simulink model "Milestone_2"  (R2020a)
settings: Solver=VariableStepAuto  StartTime=0.0  StopTime=3  RelTol=1e-3
libraries: simulink x10
settings Model: Creator=michk  LastModifiedBy=matthewterblanche

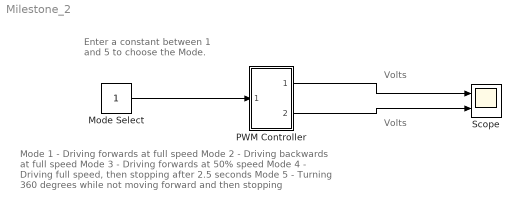
== system Milestone_2 ==
  note: Mode 1 - Driving forwards at full speed
      |
      | Mode 2 - Driving backwards at full speed
      |
      | Mode 3 - Driving forwards at 50% speed
      |
      | Mode 4 - Driving full speed, then stopping after 2.5 seconds
      |
      | Mode 5 - Turning 360 degrees while not moving forward and 			 then stopping
  note: Enter a constant between 1 and 5 to choose the Mode.
  note: Volts
  note: Volts
  Mode Select : Constant
  PWM Controller : Subsystem
  Scope : Scope  NumInputPorts=2
  wires:
  PWM Controller/2(Out2) -> Scope/2
  Mode Select/1 -> PWM Controller/1(In1)
  PWM Controller/1(Out1) -> Scope/1

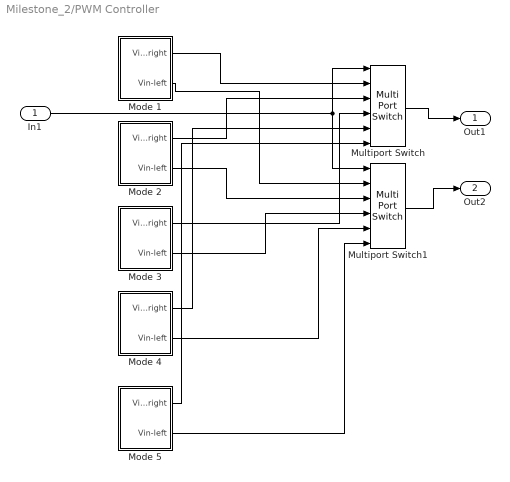
== system Milestone_2/PWM Controller ==
  In1 : Inport
  Mode 1 : Subsystem
  Mode 2 : Subsystem
  Mode 3 : Subsystem
  Mode 4 : Subsystem
  Mode 5 : Subsystem
  Multiport Switch : MultiPortSwitch  Inputs=5
  Multiport Switch1 : MultiPortSwitch  Inputs=5
  Out1 : Outport
  Out2 : Outport  Port=2
  wires:
  Multiport Switch/1 -> Out1/1
  Multiport Switch1/1 -> Out2/1
  In1/1 -> Multiport Switch/1, Multiport Switch1/1
  Mode 2/2(Vin-left) -> Multiport Switch1/3
  Mode 3/1(Vin-right) -> Multiport Switch/4
  Mode 5/2(Vin-left) -> Multiport Switch1/6
  Mode 4/1(Vin-right) -> Multiport Switch/5
  Mode 5/1(Vin-right) -> Multiport Switch/6
  Mode 2/1(Vin-right) -> Multiport Switch/3
  Mode 1/1(Vin-right) -> Multiport Switch/2
  Mode 1/2(Vin-left) -> Multiport Switch1/2
  Mode 4/2(Vin-left) -> Multiport Switch1/5
  Mode 3/2(Vin-left) -> Multiport Switch1/4

== system Milestone_2/PWM Controller/Mode 1 ==
  Subsystem : Subsystem
  Subsystem1 : Subsystem
  Vin-right : Outport
  Vin-left : Outport  Port=2
  wires:
  Subsystem1/1(Vin-left) -> Vin-left/1
  Subsystem/1(Vin-right) -> Vin-right/1

== system Milestone_2/PWM Controller/Mode 2 ==
  Subsystem : Subsystem
  Subsystem1 : Subsystem
  Vin-right : Outport
  Vin-left : Outport  Port=2
  wires:
  Subsystem1/1(Vin-left) -> Vin-left/1
  Subsystem/1(Vin-right) -> Vin-right/1

== system Milestone_2/PWM Controller/Mode 3 ==
  Subsystem : Subsystem
  Subsystem1 : Subsystem
  Vin-right : Outport
  Vin-left : Outport  Port=2
  wires:
  Subsystem1/1(Vin-left) -> Vin-left/1
  Subsystem/1(Vin-right) -> Vin-right/1

== system Milestone_2/PWM Controller/Mode 4 ==
  note: Stop motor after 2.5s
  Constant : Constant  Value=0
  Product : Product
  Product1 : Product
  Subsystem : Subsystem
  Subsystem1 : Subsystem
  Transport Delay : TransportDelay  DelayTime=2.5  InitialOutput=1  BufferSize=25600
  Vin-right : Outport
  Vin-left : Outport  Port=2
  wires:
  Subsystem1/1(Vin-left) -> Product/2
  Subsystem/1(Vin-right) -> Product1/2
  Product/1 -> Vin-left/1
  Product1/1 -> Vin-right/1
  Transport Delay/1 -> Product/1, Product1/1
  Constant/1 -> Transport Delay/1

== system Milestone_2/PWM Controller/Mode 5 ==
  Constant : Constant  Value=0
  Product : Product
  Product1 : Product
  Subsystem : Subsystem
  Subsystem1 : Subsystem
  Time motor must be on : TransportDelay  DelayTime=(0.175*pi/0.75)  InitialOutput=1  BufferSize=8192
  Vin-right : Outport
  Vin-left : Outport  Port=2
  wires:
  Constant/1 -> Time motor must be on/1
  Time motor must be on/1 -> Product1/1, Product/1
  Subsystem/1(Vin-right) -> Product/2
  Product/1 -> Vin-right/1
  Subsystem1/1(Vin-left) -> Product1/2
  Product1/1 -> Vin-left/1

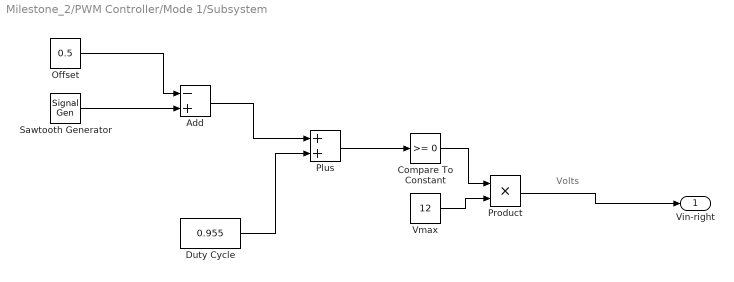
== system Milestone_2/PWM Controller/Mode 1/Subsystem ==
  note: Volts
  Add : Sum  Inputs=-+
  Compare To Constant : simulink/Logic and Bit Operations/Compare To Constant  relop=>=  const=0  OutDataTypeStr=boolean
  Duty Cycle : Constant  Value=0.955
  Offset : Constant  Value=0.5
  Plus : Sum
  Product : Product
  Sawtooth Generator : SignalGenerator  WaveForm=sawtooth  Amplitude=0.5  Frequency=10
  Vmax : Constant  Value=12
  Vin-right : Outport
  wires:
  Sawtooth Generator/1 -> Add/2
  Product/1 -> Vin-right/1
  Vmax/1 -> Product/2
  Duty Cycle/1 -> Plus/2
  Plus/1 -> Compare To Constant/1
  Offset/1 -> Add/1
  Compare To Constant/1 -> Product/1
  Add/1 -> Plus/1

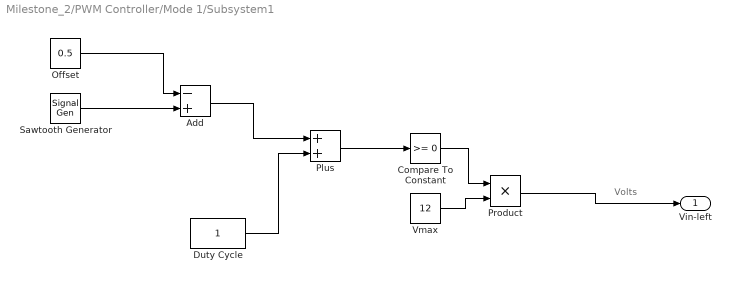
== system Milestone_2/PWM Controller/Mode 1/Subsystem1 ==
  note: Volts
  Add : Sum  Inputs=-+
  Compare To Constant : simulink/Logic and Bit Operations/Compare To Constant  relop=>=  const=0  OutDataTypeStr=boolean
  Duty Cycle : Constant
  Offset : Constant  Value=0.5
  Plus : Sum
  Product : Product
  Sawtooth Generator : SignalGenerator  WaveForm=sawtooth  Amplitude=0.5  Frequency=10
  Vmax : Constant  Value=12
  Vin-left : Outport
  wires:
  Sawtooth Generator/1 -> Add/2
  Product/1 -> Vin-left/1
  Vmax/1 -> Product/2
  Duty Cycle/1 -> Plus/2
  Plus/1 -> Compare To Constant/1
  Offset/1 -> Add/1
  Compare To Constant/1 -> Product/1
  Add/1 -> Plus/1

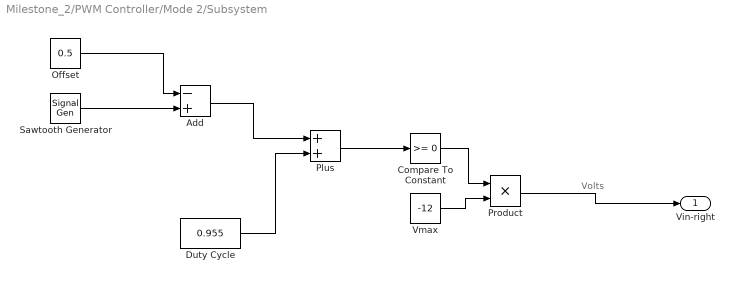
== system Milestone_2/PWM Controller/Mode 2/Subsystem ==
  note: Volts
  Add : Sum  Inputs=-+
  Compare To Constant : simulink/Logic and Bit Operations/Compare To Constant  relop=>=  const=0  OutDataTypeStr=boolean
  Duty Cycle : Constant  Value=0.955
  Offset : Constant  Value=0.5
  Plus : Sum
  Product : Product
  Sawtooth Generator : SignalGenerator  WaveForm=sawtooth  Amplitude=0.5  Frequency=10
  Vmax : Constant  Value=-12
  Vin-right : Outport
  wires:
  Sawtooth Generator/1 -> Add/2
  Product/1 -> Vin-right/1
  Vmax/1 -> Product/2
  Duty Cycle/1 -> Plus/2
  Plus/1 -> Compare To Constant/1
  Offset/1 -> Add/1
  Compare To Constant/1 -> Product/1
  Add/1 -> Plus/1

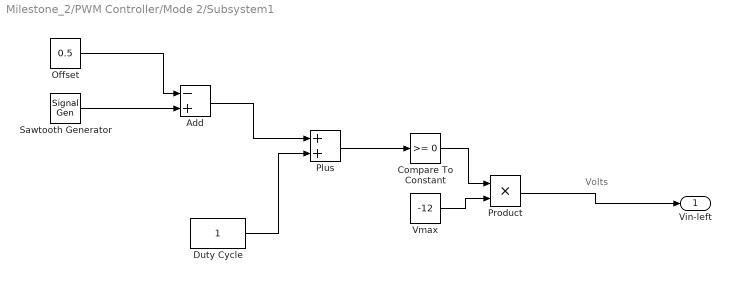
== system Milestone_2/PWM Controller/Mode 2/Subsystem1 ==
  note: Volts
  Add : Sum  Inputs=-+
  Compare To Constant : simulink/Logic and Bit Operations/Compare To Constant  relop=>=  const=0  OutDataTypeStr=boolean
  Duty Cycle : Constant
  Offset : Constant  Value=0.5
  Plus : Sum
  Product : Product
  Sawtooth Generator : SignalGenerator  WaveForm=sawtooth  Amplitude=0.5  Frequency=10
  Vmax : Constant  Value=-12
  Vin-left : Outport
  wires:
  Sawtooth Generator/1 -> Add/2
  Product/1 -> Vin-left/1
  Vmax/1 -> Product/2
  Duty Cycle/1 -> Plus/2
  Plus/1 -> Compare To Constant/1
  Offset/1 -> Add/1
  Compare To Constant/1 -> Product/1
  Add/1 -> Plus/1

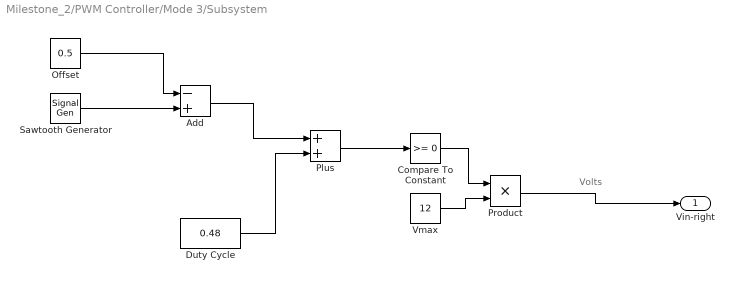
== system Milestone_2/PWM Controller/Mode 3/Subsystem ==
  note: Volts
  Add : Sum  Inputs=-+
  Compare To Constant : simulink/Logic and Bit Operations/Compare To Constant  relop=>=  const=0  OutDataTypeStr=boolean
  Duty Cycle : Constant  Value=0.48
  Offset : Constant  Value=0.5
  Plus : Sum
  Product : Product
  Sawtooth Generator : SignalGenerator  WaveForm=sawtooth  Amplitude=0.5  Frequency=10
  Vmax : Constant  Value=12
  Vin-right : Outport
  wires:
  Sawtooth Generator/1 -> Add/2
  Product/1 -> Vin-right/1
  Vmax/1 -> Product/2
  Duty Cycle/1 -> Plus/2
  Plus/1 -> Compare To Constant/1
  Offset/1 -> Add/1
  Compare To Constant/1 -> Product/1
  Add/1 -> Plus/1

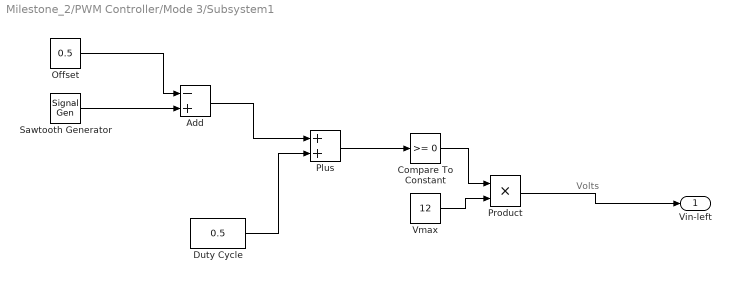
== system Milestone_2/PWM Controller/Mode 3/Subsystem1 ==
  note: Volts
  Add : Sum  Inputs=-+
  Compare To Constant : simulink/Logic and Bit Operations/Compare To Constant  relop=>=  const=0  OutDataTypeStr=boolean
  Duty Cycle : Constant  Value=0.5
  Offset : Constant  Value=0.5
  Plus : Sum
  Product : Product
  Sawtooth Generator : SignalGenerator  WaveForm=sawtooth  Amplitude=0.5  Frequency=10
  Vmax : Constant  Value=12
  Vin-left : Outport
  wires:
  Sawtooth Generator/1 -> Add/2
  Product/1 -> Vin-left/1
  Vmax/1 -> Product/2
  Duty Cycle/1 -> Plus/2
  Plus/1 -> Compare To Constant/1
  Offset/1 -> Add/1
  Compare To Constant/1 -> Product/1
  Add/1 -> Plus/1

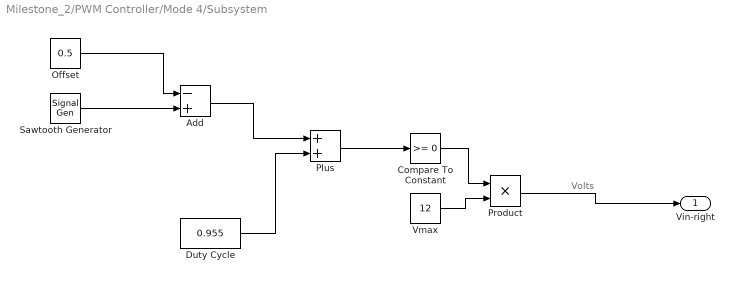
== system Milestone_2/PWM Controller/Mode 4/Subsystem ==
  note: Volts
  Add : Sum  Inputs=-+
  Compare To Constant : simulink/Logic and Bit Operations/Compare To Constant  relop=>=  const=0  OutDataTypeStr=boolean
  Duty Cycle : Constant  Value=0.955
  Offset : Constant  Value=0.5
  Plus : Sum
  Product : Product
  Sawtooth Generator : SignalGenerator  WaveForm=sawtooth  Amplitude=0.5  Frequency=10
  Vmax : Constant  Value=12
  Vin-right : Outport
  wires:
  Sawtooth Generator/1 -> Add/2
  Product/1 -> Vin-right/1
  Vmax/1 -> Product/2
  Duty Cycle/1 -> Plus/2
  Plus/1 -> Compare To Constant/1
  Offset/1 -> Add/1
  Compare To Constant/1 -> Product/1
  Add/1 -> Plus/1

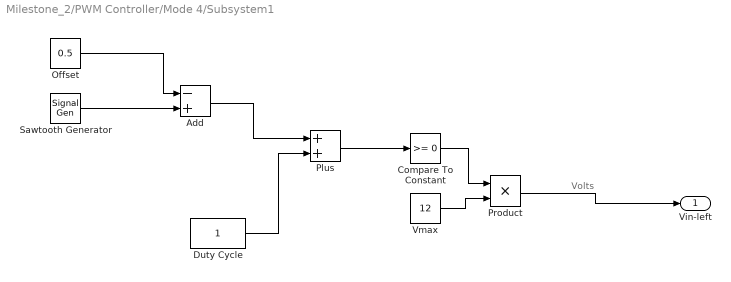
== system Milestone_2/PWM Controller/Mode 4/Subsystem1 ==
  note: Volts
  Add : Sum  Inputs=-+
  Compare To Constant : simulink/Logic and Bit Operations/Compare To Constant  relop=>=  const=0  OutDataTypeStr=boolean
  Duty Cycle : Constant
  Offset : Constant  Value=0.5
  Plus : Sum
  Product : Product
  Sawtooth Generator : SignalGenerator  WaveForm=sawtooth  Amplitude=0.5  Frequency=10
  Vmax : Constant  Value=12
  Vin-left : Outport
  wires:
  Sawtooth Generator/1 -> Add/2
  Product/1 -> Vin-left/1
  Vmax/1 -> Product/2
  Duty Cycle/1 -> Plus/2
  Plus/1 -> Compare To Constant/1
  Offset/1 -> Add/1
  Compare To Constant/1 -> Product/1
  Add/1 -> Plus/1

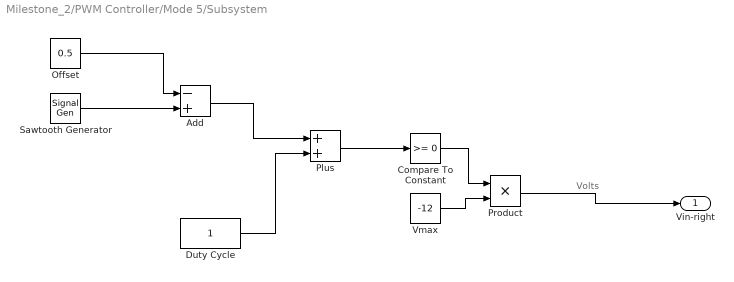
== system Milestone_2/PWM Controller/Mode 5/Subsystem ==
  note: Volts
  Add : Sum  Inputs=-+
  Compare To Constant : simulink/Logic and Bit Operations/Compare To Constant  relop=>=  const=0  OutDataTypeStr=boolean
  Duty Cycle : Constant
  Offset : Constant  Value=0.5
  Plus : Sum
  Product : Product
  Sawtooth Generator : SignalGenerator  WaveForm=sawtooth  Amplitude=0.5  Frequency=10
  Vmax : Constant  Value=-12
  Vin-right : Outport
  wires:
  Sawtooth Generator/1 -> Add/2
  Product/1 -> Vin-right/1
  Vmax/1 -> Product/2
  Duty Cycle/1 -> Plus/2
  Plus/1 -> Compare To Constant/1
  Offset/1 -> Add/1
  Compare To Constant/1 -> Product/1
  Add/1 -> Plus/1

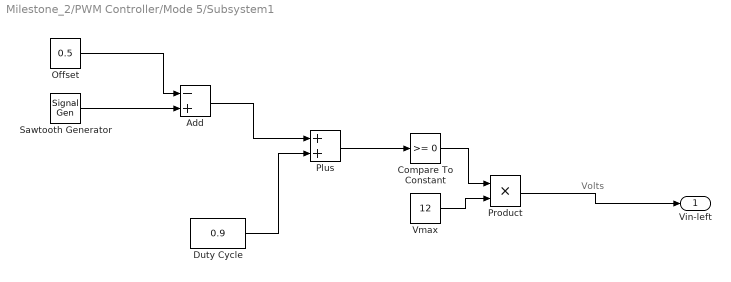
== system Milestone_2/PWM Controller/Mode 5/Subsystem1 ==
  note: Volts
  Add : Sum  Inputs=-+
  Compare To Constant : simulink/Logic and Bit Operations/Compare To Constant  relop=>=  const=0  OutDataTypeStr=boolean
  Duty Cycle : Constant  Value=0.9
  Offset : Constant  Value=0.5
  Plus : Sum
  Product : Product
  Sawtooth Generator : SignalGenerator  WaveForm=sawtooth  Amplitude=0.5  Frequency=10
  Vmax : Constant  Value=12
  Vin-left : Outport
  wires:
  Sawtooth Generator/1 -> Add/2
  Product/1 -> Vin-left/1
  Vmax/1 -> Product/2
  Duty Cycle/1 -> Plus/2
  Plus/1 -> Compare To Constant/1
  Offset/1 -> Add/1
  Compare To Constant/1 -> Product/1
  Add/1 -> Plus/1
